simulink model "Laengsdynamik"  (R2019a)
settings: Solver=ode4  StartTime=0.0  StopTime=10.0  FixedStep=0.001  RelTol=1e-3
model workspace (MAT data in the model file):
  FBv = [-0.360628002737 -0.359628002737 -0.358628002737 -0.357628002737 -0.356628002737 -0.355628002737 -0.354628002737 -0.353628002737 -0.352628002737 -0.351628002737 -0.350628002737 -0.349628002737 ... (3119 elements, 1x3119)]
  G_g = 16.59
  G_h = 8.17
  g = 9.81
  h_s = 0.5
  l = 2.8
  l_v = 1.344
  reifenX = [0 0.25 1]
  reifenY = [0 1 1]
  useController = 1
  v0 = 22.2222222222
  z_time = [0 1.5 1.95 2.15 10]
  z_vals = [0 0 0.1 1 1]
  zh_z = 1
  zv_z = 1
libraries: simulink x3
(part 2 of 2)

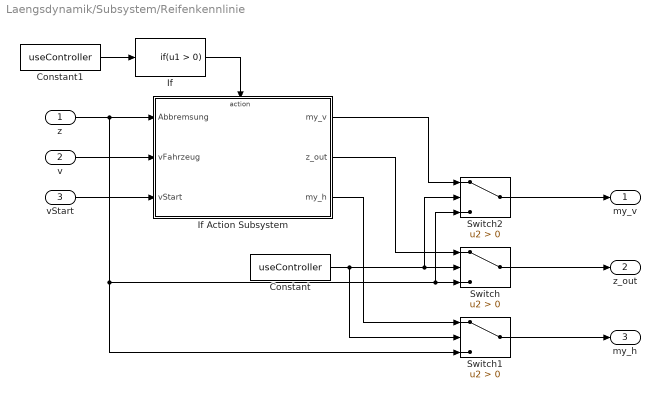
== system Laengsdynamik/Subsystem/Reifenkennlinie ==
  z : Inport
  v : Inport  Port=2
  vStart : Inport  Port=3
  Constant : Constant  Value=useController
  Constant1 : Constant  Value=useController
  If : If  ShowElse=off
  If Action Subsystem : Subsystem  TreatAsAtomicUnit=on
  Switch : Switch  Criteria=u2 > Threshold
  Switch1 : Switch  Criteria=u2 > Threshold
  Switch2 : Switch  Criteria=u2 > Threshold
  my_v : Outport
  z_out : Outport  Port=2
  my_h : Outport  Port=3
  wires:
  z/1 -> Switch1/3, Switch2/3, Switch/3, If Action Subsystem/1(Abbremsung)
  v/1 -> If Action Subsystem/2(vFahrzeug)
  vStart/1 -> If Action Subsystem/3(vStart)
  Constant/1 -> Switch1/2, Switch2/2, Switch/2
  If Action Subsystem/2(z_out) -> Switch/1
  Switch/1 -> z_out/1
  Switch1/1 -> my_h/1
  If Action Subsystem/3(my_h) -> Switch1/1
  Switch2/1 -> my_v/1
  If Action Subsystem/1(my_v) -> Switch2/1
  Constant1/1 -> If/1
  If/1 -> If Action Subsystem/Action

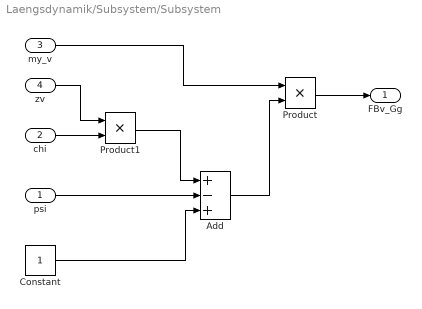
== system Laengsdynamik/Subsystem/Subsystem ==
  psi : Inport
  chi : Inport  Port=2
  my_v : Inport  Port=3
  zv : Inport  Port=4
  Add : Sum  Inputs=+-+
  Constant : Constant
  Product : Product
  Product1 : Product
  FBv_Gg : Outport
  wires:
  zv/1 -> Product1/1
  Product/1 -> FBv_Gg/1
  chi/1 -> Product1/2
  Product1/1 -> Add/1
  psi/1 -> Add/2
  Constant/1 -> Add/3
  Add/1 -> Product/2
  my_v/1 -> Product/1

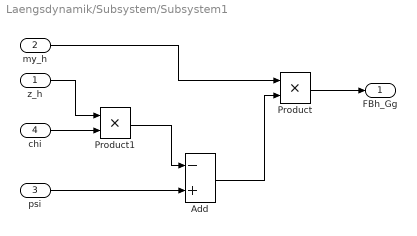
== system Laengsdynamik/Subsystem/Subsystem1 ==
  z_h : Inport
  my_h : Inport  Port=2
  psi : Inport  Port=3
  chi : Inport  Port=4
  Add : Sum  Inputs=-+
  Product : Product
  Product1 : Product
  FBh_Gg : Outport
  wires:
  z_h/1 -> Product1/1
  Product/1 -> FBh_Gg/1
  chi/1 -> Product1/2
  Product1/1 -> Add/1
  psi/1 -> Add/2
  Add/1 -> Product/2
  my_h/1 -> Product/1

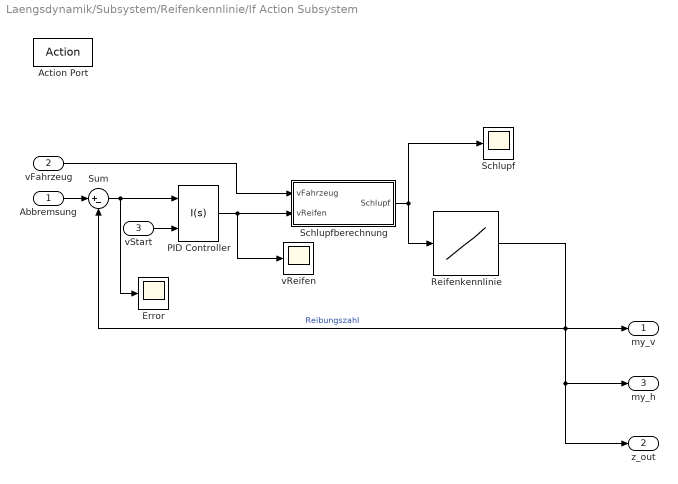
== system Laengsdynamik/Subsystem/Reifenkennlinie/If Action Subsystem ==
  Abbremsung : Inport
  vFahrzeug : Inport  Port=2
  vStart : Inport  Port=3
  Action Port : ActionPort  ActionPortLabel=if { }
  Error : Scope
  PID Controller : simulink/Continuous/PID Controller  Controller=I  Form=Parallel  TimeDomain=Continuous-time  SampleTime=-1  IntegratorMethod=Forward Euler  FilterMethod=Forward Euler  ControllerParametersSource=internal  P=0  I=-700  D=0  UseFilter=on  N=100  TunerSelectOption=Transfer Function Based (PID Tuner App)  InitialConditionSource=external  InitialConditionForIntegrator=0  InitialConditionForFilter=0  DifferentiatorICPrevScaledInput=0  ExternalReset=none  TrackingMode=off  Kt=1  LimitOutput=off  UpperSaturationLimit=inf  LowerSaturationLimit=-inf  LinearizeAsGain=on  AntiWindupMode=none  Kb=1  POutMin=[]  POutMax=[]  IOutMin=[]  IOutMax=[]  DOutMin=[]  DOutMax=[]  NOutMin=[]  NOutMax=[]  SumOutMin=[]  SumOutMax=[]  SaturationOutMin=[]  SaturationOutMax=[]  PParamMin=[]  PParamMax=[]  IParamMin=[]  IParamMax=[]  DParamMin=[]  DParamMax=[]  NParamMin=[]  NParamMax=[]  KbParamMin=[]  KbParamMax=[]  KtParamMin=[]  KtParamMax=[]  KbOutMin=[]  KbOutMax=[]  KtOutMin=[]  KtOutMax=[]  IntegratorOutMin=[]  IntegratorOutMax=[]  FilterOutMin=[]  FilterOutMax=[]  SumI1OutMin=[]  SumI1OutMax=[]  SumI2OutMin=[]  SumI2OutMax=[]  SumI3OutMin=[]  SumI3OutMax=[]  SumI4OutMin=[]  SumI4OutMax=[]  SumDOutMin=[]  SumDOutMax=[]  DifferentiatorOutMin=[]  DifferentiatorOutMax=[]  FilterDiffOutCoefMin=[]  FilterDiffOutCoefMax=[]  ReciprocalOutMin=[]  ReciprocalOutMax=[]  SumDenOutMin=[]  SumDenOutMax=[]  SumNumOutMin=[]  SumNumOutMax=[]  DivideOutMin=[]  DivideOutMax=[]  IntegratorContinuousStateAttributes=''  IntegratorStateMustResolveToSignalObject=off  IntegratorRTWStateStorageClass=Auto  FilterContinuousStateAttributes=''  FilterStateMustResolveToSignalObject=off  FilterRTWStateStorageClass=Auto  ParallelPVariant=Disabled  IdealPVariant=Disabled  IVariant=InternalParameters  DVariant=Disabled  IntegratorVariant=Continuous  SatVariant=Disabled  AWVariant=Passthrough  PCopyVariant=Disabled  TRVariant=Disabled  FdbkBlocksVariant=Forward  IdealPFdbkVariant=Disabled  SatFdbkVariant=Disabled  DerivativeFilterVariant=Disabled  NVariant=Disabled  NCopyVariant=Disabled_SignalSpec  FilterICVariant=Disabled  IntegratorICVariant=ExternalICs  ExternalResetVariant=Disabled  TRSumVariant=Passthrough  SumFdbkVariant=Disabled  SumVariant=Passthrough_I
  Reifenkennlinie : Lookup_n-D  NumberOfTableDimensions=1  BreakpointsForDimension1=reifenX  Table=reifenY  ExtrapMethod=Clip  UseLastTableValue=on  InternalRulePriority=Speed  RndMeth=Simplest  InputSameDT=on
  Schlupf : Scope
  Schlupfberechnung : Subsystem
  Sum : Sum  Inputs=|+-
  vReifen : Scope
  my_v : Outport
  z_out : Outport  Port=2
  my_h : Outport  Port=3
  wires:
  Abbremsung/1 -> Sum/1
  PID Controller/1 -> vReifen/1, Schlupfberechnung/2(vReifen)
  vStart/1 -> PID Controller/2
  Schlupfberechnung/1(Schlupf) -> Schlupf/1, Reifenkennlinie/1
  Reifenkennlinie/1 -> Sum/2, my_h/1, z_out/1, my_v/1  "Reibungszahl"
  vFahrzeug/1 -> Schlupfberechnung/1(vFahrzeug)
  Sum/1 -> PID Controller/1, Error/1

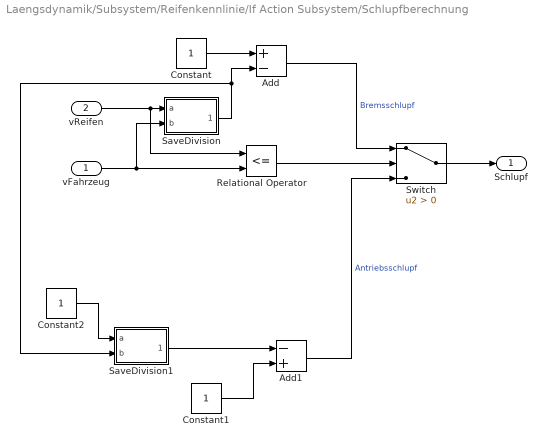
== system Laengsdynamik/Subsystem/Reifenkennlinie/If Action Subsystem/Schlupfberechnung ==
  vFahrzeug : Inport
  vReifen : Inport  Port=2
  Add : Sum  Inputs=+-
  Add1 : Sum  Inputs=-+
  Constant : Constant
  Constant1 : Constant
  Constant2 : Constant
  Relational Operator : RelationalOperator  Operator=<=  OutDataTypeStr=boolean  RndMeth=Simplest
  SaveDivision : Subsystem
  SaveDivision1 : Subsystem
  Switch : Switch  Criteria=u2 > Threshold
  Schlupf : Outport
  wires:
  Constant/1 -> Add/1
  vFahrzeug/1 -> SaveDivision/2(b), Relational Operator/2
  SaveDivision/1(division) -> SaveDivision1/2(b), Add/2
  Switch/1 -> Schlupf/1
  Add/1 -> Switch/1  "Bremsschlupf"
  vReifen/1 -> SaveDivision/1(a), Relational Operator/1
  Relational Operator/1 -> Switch/2
  Constant1/1 -> Add1/2
  Add1/1 -> Switch/3  "Antriebsschlupf"
  SaveDivision1/1(division) -> Add1/1
  Constant2/1 -> SaveDivision1/1(a)

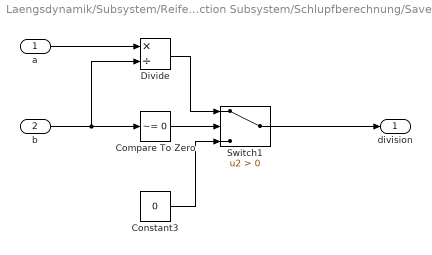
== system Laengsdynamik/Subsystem/Reifenkennlinie/If Action Subsystem/Schlupfberechnung/SaveDivision ==
  a : Inport
  b : Inport  Port=2
  Compare To Zero : simulink/Logic and Bit Operations/Compare To Zero  relop=~=  OutDataTypeStr=boolean
  Constant3 : Constant  Value=0
  Divide : Product  Inputs=*/
  Switch1 : Switch  Criteria=u2 > Threshold
  division : Outport
  wires:
  Switch1/1 -> division/1
  Divide/1 -> Switch1/1
  Compare To Zero/1 -> Switch1/2
  Constant3/1 -> Switch1/3
  b/1 -> Divide/2, Compare To Zero/1
  a/1 -> Divide/1

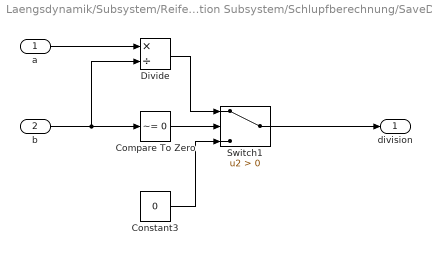
== system Laengsdynamik/Subsystem/Reifenkennlinie/If Action Subsystem/Schlupfberechnung/SaveDivision1 ==
  a : Inport
  b : Inport  Port=2
  Compare To Zero : simulink/Logic and Bit Operations/Compare To Zero  relop=~=  OutDataTypeStr=boolean
  Constant3 : Constant  Value=0
  Divide : Product  Inputs=*/
  Switch1 : Switch  Criteria=u2 > Threshold
  division : Outport
  wires:
  Switch1/1 -> division/1
  Divide/1 -> Switch1/1
  Compare To Zero/1 -> Switch1/2
  Constant3/1 -> Switch1/3
  b/1 -> Divide/2, Compare To Zero/1
  a/1 -> Divide/1
